simulink model "dbaSimRasp"  (R2020b)
settings: Solver=FixedStepAuto  StartTime=0.0  StopTime=inf  RelTol=1e-3  EnableMultiTasking=on
model workspace (MAT data in the model file):
  Fs = Simulink.Parameter
  Fs.Value = 44100
  Fs.DataType = 'auto'
  Fs.Dimensions = [1 1]
  N = Simulink.Parameter
  N.Value = 32768
  N.DataType = 'auto'
  N.Dimensions = [1 1]
  x = Simulink.Parameter
  x.Value = [-1 -1]
  x.DataType = 'auto'
  x.Dimensions = [1 2]
undefined symbols (not defined in the file): hw
libraries: raspberrypiIOTlib x2, embdlinuxlib x1, dspspect3 x1, audiofilters x1, dspsigops x1
settings Model: SimulationMode=external  OrderedModelArguments=off  Creator=oskar  LastModifiedBy=oskar
settings SolverCC: PositivePriorityOrder=on  AutoInsertRateTranBlk=on
settings OptimizationCC: EnhancedBackFolding=on  PassReuseOutputArgsAs=Individual arguments  ZeroExternalMemoryAtStartup=off  ZeroInternalMemoryAtStartup=off  MaxStackSize=64  OptimizeBlockOrder=speed  DifferentSizesBufferReuse=on  OptimizationCustomize=off  EfficientTunableParamExpr=on
settings DebuggingCC: ParameterTunabilityLossMsg=error
settings HardwareCC: ProdBitPerPointer=32  ProdBitPerSizeT=32  ProdBitPerPtrDiffT=32  ProdLargestAtomicInteger=Long  ProdLargestAtomicFloat=Double  ProdWordSize=32  ProdLongLongMode=on  ProdHWDeviceType=ARM Compatible->ARM Cortex
settings RTWCC: Description=Embedded Coder  SystemTargetFile=ert.tlc  HardwareBoard=Raspberry Pi  TLCOptions="-aInlineSetEventsForThisBaseRateFcn=TLC_FALSE -aSuppressMultiTaskScheduler=TLC_FALSE  -aRateBasedStepFcn=0"  TemplateMakefile=ert_default_tmf  Toolchain=GNU GCC Raspberry Pi  BuildConfiguration=Faster Runs
settings CodeAppCC: ForceParamTrailComments=on  IgnoreCustomStorageClasses=off  OperatorAnnotations=on  SimulinkDataObjDesc=on  SFDataObjDesc=on  InsertBlockDesc=on
settings ERTTargetCC: SupportVariableSizeSignals=on  ExtMode=on  ExtModeTransport=2  ExtModeStaticAlloc=on  ExtModeMexFile=ext_xcp  ExtModeMexArgs='10.50.74.8' 0 17725  ExtModeIntrfLevel=Level2 - Open

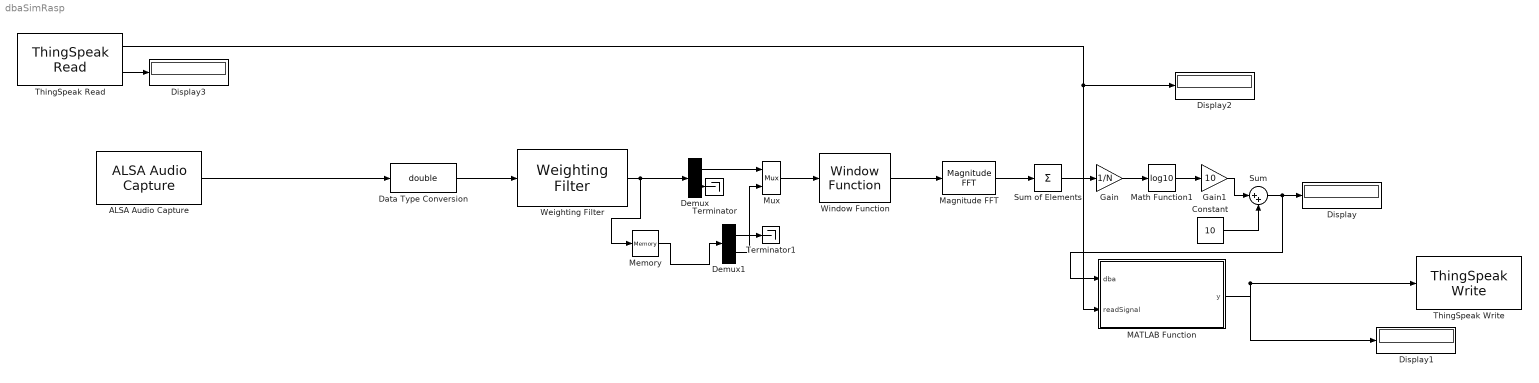
== system dbaSimRasp ==
  ALSA Audio Capture : embdlinuxlib/ALSA Audio Capture  deviceStr=hw:2,0  DataBitDepth=16-bit integer  numberOfChannels=1  sampleRateEnum=48000  frameSize=4800  QueueDuration=0.5  blockPlatform=RASPBERRYPI
      settings: SourceProductBaseCode=SC_BEAGLEBONE_BLUE,NVIDIA,RASPPI
  Constant : Constant  Value=10
  Data Type Conversion : DataTypeConversion  OutDataTypeStr=double  RndMeth=Nearest  SaturateOnIntegerOverflow=on
  Demux : Demux  Outputs=x
  Demux1 : Demux  Outputs=x
  Display{,1..3} (4 alike) : Display
  Gain : Gain  Gain=1/N
  Gain1 : Gain  Gain=10
  MATLAB Function : MATLAB Function  TreatAsAtomicUnit=on
  Magnitude FFT : dspspect3/Magnitude FFT  mag_or_magsq=Magnitude squared  FFTImplementation=Auto  fftLenInherit=off  fftsize=32768  WrapInput=on
      settings: SourceProductName=DSP System Toolbox
  Math Function1 : Math  Operator=log10  SaturateOnIntegerOverflow=on
  Memory : Memory
  Mux : Mux  Inputs=2
  Sum : Sum  Inputs=|++
  Sum of Elements : Sum  Inputs=+
  Terminator : Terminator
  Terminator1 : Terminator
  ThingSpeak Read : raspberrypiIOTlib/ThingSpeak Read  ChannelID=1959854  ChannelAccess=Private  ReadAPIKey=I25N4WEBXG99TXVO  FieldNumber=1  PrintDiagnosticMessages=on  SampleTime=15
      settings: SourceProductBaseCode=RASPPI
  ThingSpeak Write : raspberrypiIOTlib/ThingSpeak Write  UpdateURL=https://api.thingspeak.com/update  WriteAPIKey=5IVATAVA6XG7PI2I  NumberOfFields=1  UpdateInterval=15  PrintDiagnosticMessages=on  CoordinatesEnabled=off  CoordSrc=Block dialog  Coordinates=[42.29971, -71.350719, 69.29]  blockPlatform=Raspberry Pi
      settings: SourceProductBaseCode=RASPPI
  Weighting Filter : audiofilters/Weighting Filter  Method=A-weighting  InheritSampleRate=on  SampleRate=44100  SimulateUsing=Code generation  MaskClassType=No mask
      settings: SourceProductBaseCode=AU
  Window Function : dspsigops/Window Function  winmode=Apply window to input  wintype=Kaiser  sampmode=Continuous  samptime=1  N=64  Rs=50  beta=5  winsamp=Symmetric  UserWindow=hamming  OptParams=off  UserParams={'symmetric'}  dataType=double  isSigned=on  wordLen=16  udDataType=sfix(16)  fracBitsMode=Best precision  numFracBits=15  roundingMode=Floor  overflowMode=off  numSidelobes=4  sidelobeLevel=-30
      settings: SourceProductBaseCode=DS
  wires:
  Data Type Conversion/1 -> Weighting Filter/1
  Weighting Filter/1 -> Memory/1, Demux/1
  Mux/1 -> Window Function/1
  Demux/1 -> Mux/1
  Memory/1 -> Demux1/1
  Demux1/2 -> Mux/2
  Window Function/1 -> Magnitude FFT/1
  Magnitude FFT/1 -> Sum of Elements/1
  Sum of Elements/1 -> Gain/1
  Gain/1 -> Math Function1/1
  Math Function1/1 -> Gain1/1
  Gain1/1 -> Sum/1
  Constant/1 -> Sum/2
  Sum/1 -> MATLAB Function/1(dba), Display/1
  Demux/2 -> Terminator/1
  ALSA Audio Capture/1 -> Data Type Conversion/1
  ThingSpeak Read/2 -> Display3/1
  MATLAB Function/1(y) -> ThingSpeak Write/1, Display1/1
  Demux1/1 -> Terminator1/1
  ThingSpeak Read/1 -> MATLAB Function/2(readSignal), Display2/1

== matlab function dbaSimRasp/MATLAB Function ==
  data: dba input; y output; readSignal input
function y = fcn(dba, readSignal)
    if (readSignal >= 70)
        y = dba;
    else
        y = NaN;
    end
end
